simulink model "fblin_singletrack_schlacher"  (R2021a)
settings: Solver=ode45  StartTime=0.0  StopTime=20  RelTol=1e-3
PostLoadFcn:
  | clear all;
  | 
  | lf  = 0.1368;
  | lr  = 0.1232;
  | m  = 1.9;
  | mu = 0.385;
  | Cf = 50.13;
  | Cr = 122.05;
  | J = 0.029;
  | 
  | V0 = 1;
  | Vxp0 = 1;
  | Vxpf = 5;
  | Vyp0 = 0;
  | Vypf = 1;
settings Model: Creator=l_lan  LastModifiedBy=bascetta
settings SolverCC: MaxConsecutiveZCs=10000  MaxConsecutiveMinStep=1000
settings DataIOCC: SaveOutput=off  SignalLogging=off  DSMLogging=off  SaveTime=off  ReturnWorkspaceOutputs=off

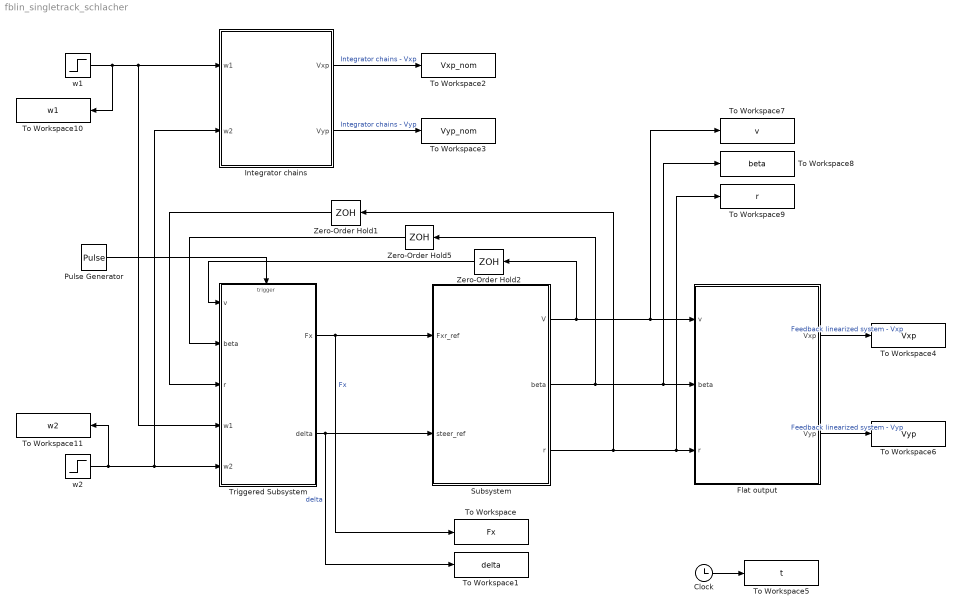
== system fblin_singletrack_schlacher ==
  Clock : Clock
  Flat output : Subsystem
  Integrator chains : Subsystem
  Pulse Generator : DiscretePulseGenerator  PulseType=Time based  Period=0.01  PulseWidth=50
  Subsystem : Subsystem
  To Workspace : ToWorkspace  VariableName=Fx  SampleTime=0.001
      settings: Save2DSignal=2-D array (concatenate along first dimension)
  To Workspace1 : ToWorkspace  VariableName=delta  SampleTime=0.001
      settings: Save2DSignal=2-D array (concatenate along first dimension)
  To Workspace10 : ToWorkspace  VariableName=w1  SampleTime=0.001
      settings: Save2DSignal=2-D array (concatenate along first dimension)
  To Workspace11 : ToWorkspace  VariableName=w2  SampleTime=0.001
      settings: Save2DSignal=2-D array (concatenate along first dimension)
  To Workspace2 : ToWorkspace  VariableName=Vxp_nom  SampleTime=0.001
      settings: Save2DSignal=2-D array (concatenate along first dimension)
  To Workspace3 : ToWorkspace  VariableName=Vyp_nom  SampleTime=0.001
      settings: Save2DSignal=2-D array (concatenate along first dimension)
  To Workspace4 : ToWorkspace  VariableName=Vxp  SampleTime=0.001
      settings: Save2DSignal=2-D array (concatenate along first dimension)
  To Workspace5 : ToWorkspace  VariableName=t  SampleTime=0.001
      settings: Save2DSignal=2-D array (concatenate along first dimension)
  To Workspace6 : ToWorkspace  VariableName=Vyp  SampleTime=0.001
      settings: Save2DSignal=2-D array (concatenate along first dimension)
  To Workspace7 : ToWorkspace  VariableName=v  SampleTime=0.001
      settings: Save2DSignal=2-D array (concatenate along first dimension)
  To Workspace8 : ToWorkspace  VariableName=beta  SampleTime=0.001
      settings: Save2DSignal=2-D array (concatenate along first dimension)
  To Workspace9 : ToWorkspace  VariableName=r  SampleTime=0.001
      settings: Save2DSignal=2-D array (concatenate along first dimension)
  Triggered Subsystem : Subsystem  TreatAsAtomicUnit=on
  Zero-Order Hold1 : ZeroOrderHold  SampleTime=0.01
  Zero-Order Hold2 : ZeroOrderHold  SampleTime=0.01
  Zero-Order Hold5 : ZeroOrderHold  SampleTime=0.01
  w1 : Step  Before=Vxp0  After=Vxpf  SampleTime=0
  w2 : Step  Time=5  Before=Vyp0  After=Vypf  SampleTime=0
  wires:
  Subsystem/3(r) -> Flat output/3(r), To Workspace9/1, Zero-Order Hold1/1
  Integrator chains/1(Vxp) -> To Workspace2/1  "Integrator chains - Vxp"
  w1/1 -> To Workspace10/1, Triggered Subsystem/4(w1), Integrator chains/1(w1)
  w2/1 -> To Workspace11/1, Integrator chains/2(w2), Triggered Subsystem/5(w2)
  Flat output/2(Vyp) -> To Workspace6/1  "Feedback linearized system - Vyp"
  Integrator chains/2(Vyp) -> To Workspace3/1  "Integrator chains - Vyp"
  Flat output/1(Vxp) -> To Workspace4/1  "Feedback linearized system - Vxp"
  Clock/1 -> To Workspace5/1
  Subsystem/2(beta) -> Zero-Order Hold5/1, Flat output/2(beta), To Workspace8/1
  Pulse Generator/1 -> Triggered Subsystem/Trigger
  Triggered Subsystem/1(Fx) -> Subsystem/1(Fxr_ref), To Workspace/1  "Fx"
  Triggered Subsystem/2(delta) -> Subsystem/2(steer_ref), To Workspace1/1  "delta"
  Zero-Order Hold1/1 -> Triggered Subsystem/3(r)
  Zero-Order Hold2/1 -> Triggered Subsystem/1(v)
  Zero-Order Hold5/1 -> Triggered Subsystem/2(beta)
  Subsystem/1(V) -> To Workspace7/1, Flat output/1(v), Zero-Order Hold2/1

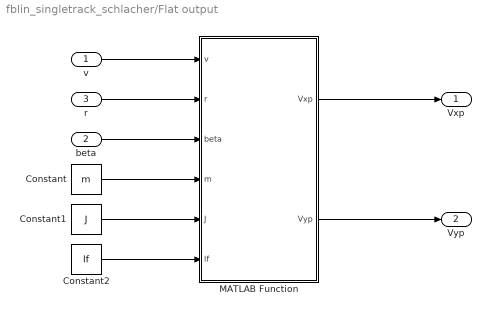
== system fblin_singletrack_schlacher/Flat output ==
  v : Inport
  beta : Inport  Port=2
  r : Inport  Port=3
  Constant : Constant  Value=m
  Constant1 : Constant  Value=J
  Constant2 : Constant  Value=lf
  MATLAB Function : MATLAB Function  TreatAsAtomicUnit=on
  Vxp : Outport
  Vyp : Outport  Port=2
  wires:
  beta/1 -> MATLAB Function/3(beta)
  r/1 -> MATLAB Function/2(r)
  v/1 -> MATLAB Function/1(v)
  Constant1/1 -> MATLAB Function/5(J)
  Constant/1 -> MATLAB Function/4(m)
  Constant2/1 -> MATLAB Function/6(lf)
  MATLAB Function/2(Vyp) -> Vyp/1
  MATLAB Function/1(Vxp) -> Vxp/1

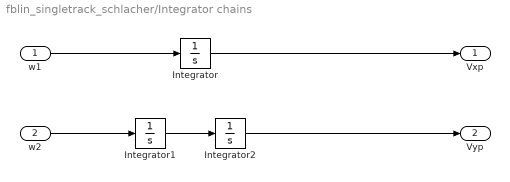
== system fblin_singletrack_schlacher/Integrator chains ==
  w1 : Inport
  w2 : Inport  Port=2
  Integrator : Integrator  InitialCondition=V0
  Integrator1 : Integrator
  Integrator2 : Integrator
  Vxp : Outport
  Vyp : Outport  Port=2
  wires:
  Integrator/1 -> Vxp/1
  Integrator1/1 -> Integrator2/1
  Integrator2/1 -> Vyp/1
  w2/1 -> Integrator1/1
  w1/1 -> Integrator/1

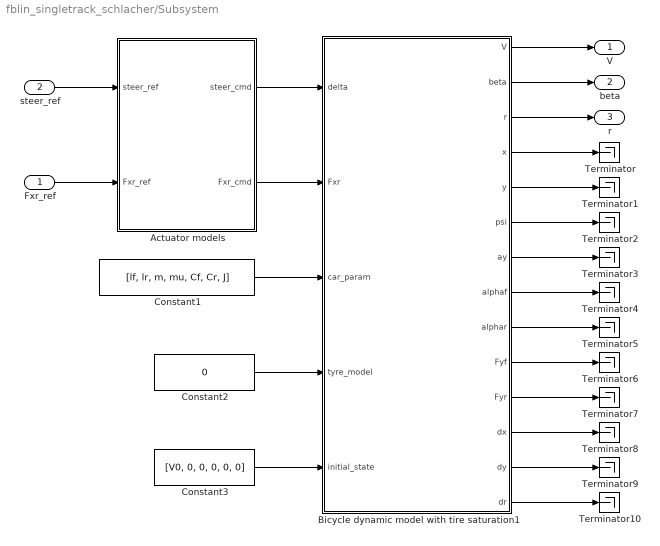
== system fblin_singletrack_schlacher/Subsystem ==
  Fxr_ref : Inport
  steer_ref : Inport  Port=2
  Actuator models : Subsystem  mask{mu_steer=1.0, wn_steer=87.62, csi_steer=0.75, tau_steer=0.055, steer_initial=0.0, mu_force=5.1282, wn_force=1000, csi_force=0.9, tau_force=0.0001, force_initial=0}
      mask prompts: mu_steer "Gain"; wn_steer "Natural frequency"; csi_steer "Damping"; tau_steer "Delay"; steer_initial "Initial value"; mu_force "Gain"; wn_force "Natural frequency"; csi_force "Damping"; tau_force "Delay"; force_initial "Initial value"
      mask DialogControl Container3 Prompt: Steer actuator parameters
      mask DialogControl Container4 Prompt: Speed actuator parameters
  Bicycle dynamic model with tire saturation1 : Subsystem
  Constant1 : Constant  Value=[lf, lr, m, mu, Cf, Cr, J]
  Constant2 : Constant  Value=0
  Constant3 : Constant  Value=[V0, 0, 0, 0, 0, 0]
  Terminator{,1..10} (11 alike) : Terminator
  V : Outport
  beta : Outport  Port=2
  r : Outport  Port=3
  wires:
  Constant2/1 -> Bicycle dynamic model with tire saturation1/4(tyre_model)
  Constant1/1 -> Bicycle dynamic model with tire saturation1/3(car_param)
  steer_ref/1 -> Actuator models/1(steer_ref)
  Actuator models/2(Fxr_cmd) -> Bicycle dynamic model with tire saturation1/2(Fxr)
  Fxr_ref/1 -> Actuator models/2(Fxr_ref)
  Actuator models/1(steer_cmd) -> Bicycle dynamic model with tire saturation1/1(delta)
  Constant3/1 -> Bicycle dynamic model with tire saturation1/5("initial_state ")
  Bicycle dynamic model with tire saturation1/3(r) -> r/1
  Bicycle dynamic model with tire saturation1/2(beta) -> beta/1
  Bicycle dynamic model with tire saturation1/1(V) -> V/1
  Bicycle dynamic model with tire saturation1/4(x) -> Terminator/1
  Bicycle dynamic model with tire saturation1/5(y) -> Terminator1/1
  Bicycle dynamic model with tire saturation1/6(psi) -> Terminator2/1
  Bicycle dynamic model with tire saturation1/7(ay) -> Terminator3/1
  Bicycle dynamic model with tire saturation1/8(alphaf) -> Terminator4/1
  Bicycle dynamic model with tire saturation1/9(alphar) -> Terminator5/1
  Bicycle dynamic model with tire saturation1/10(Fyf) -> Terminator6/1
  Bicycle dynamic model with tire saturation1/11(Fyr) -> Terminator7/1
  Bicycle dynamic model with tire saturation1/12(dx) -> Terminator8/1
  Bicycle dynamic model with tire saturation1/13(dy) -> Terminator9/1
  Bicycle dynamic model with tire saturation1/14(dr) -> Terminator10/1

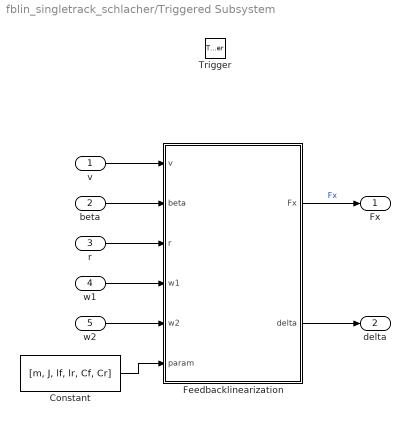
== system fblin_singletrack_schlacher/Triggered Subsystem ==
  v : Inport
  beta : Inport  Port=2
  r : Inport  Port=3
  w1 : Inport  Port=4
  w2 : Inport  Port=5
  Trigger : TriggerPort  VariantControl=(inherit)
  Constant : Constant  Value=[m, J, lf, lr, Cf, Cr]
  Feedbacklinearization : MATLAB Function  TreatAsAtomicUnit=on
  Fx : Outport
  delta : Outport  Port=2
  wires:
  Constant/1 -> Feedbacklinearization/6(param)
  v/1 -> Feedbacklinearization/1(v)
  beta/1 -> Feedbacklinearization/2(beta)
  r/1 -> Feedbacklinearization/3(r)
  w1/1 -> Feedbacklinearization/4(w1)
  w2/1 -> Feedbacklinearization/5(w2)
  Feedbacklinearization/2(delta) -> delta/1
  Feedbacklinearization/1(Fx) -> Fx/1  "Fx"

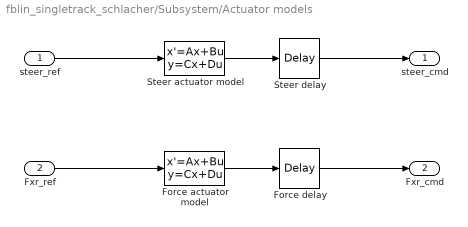
== system fblin_singletrack_schlacher/Subsystem/Actuator models ==
  steer_ref : Inport
  Fxr_ref : Inport  Port=2
  Force actuator model : StateSpace  A=[0, 1; -wn_force^2, -2*csi_force*wn_force]  B=[0; mu_force*wn_force^2]  C=[1, 0]  D=0  InitialCondition=[force_initial, 0]
  Force delay : TransportDelay  DelayTime=tau_force  InitialOutput=force_initial
  Steer actuator model : StateSpace  A=[0, 1; -wn_steer^2, -2*csi_steer*wn_steer]  B=[0; mu_steer*wn_steer^2]  C=[1, 0]  D=0  InitialCondition=[steer_initial, 0]
  Steer delay : TransportDelay  DelayTime=tau_steer  InitialOutput=steer_initial
  steer_cmd : Outport
  Fxr_cmd : Outport  Port=2
  wires:
  Fxr_ref/1 -> Force actuator model/1
  Steer actuator model/1 -> Steer delay/1
  Force actuator model/1 -> Force delay/1
  steer_ref/1 -> Steer actuator model/1
  Steer delay/1 -> steer_cmd/1
  Force delay/1 -> Fxr_cmd/1

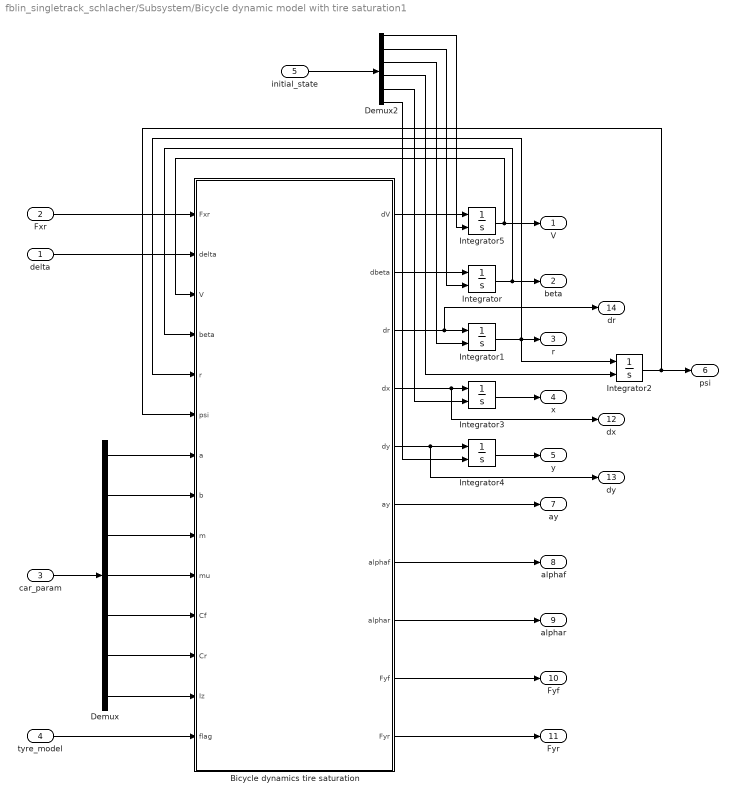
== system fblin_singletrack_schlacher/Subsystem/Bicycle dynamic model with tire saturation1 ==
  delta : Inport
  Fxr : Inport  Port=2
  car_param : Inport  Port=3
  tyre_model : Inport  Port=4
  "initial_state " : Inport  Port=5
  Bicycle dynamics tire saturation : MATLAB Function  TreatAsAtomicUnit=on
  Demux : Demux  Outputs=7
  Demux2 : Demux  Outputs=6
  Integrator{,1..5} (6 alike) : Integrator  InitialConditionSource=external
  V : Outport
  beta : Outport  Port=2
  r : Outport  Port=3
  x : Outport  Port=4
  y : Outport  Port=5
  psi : Outport  Port=6
  ay : Outport  Port=7
  alphaf : Outport  Port=8
  alphar : Outport  Port=9
  Fyf : Outport  Port=10
  Fyr : Outport  Port=11
  dx : Outport  Port=12
  dy : Outport  Port=13
  dr : Outport  Port=14
  wires:
  Fxr/1 -> Bicycle dynamics tire saturation/1(Fxr)
  delta/1 -> Bicycle dynamics tire saturation/2(delta)
  Bicycle dynamics tire saturation/2(dbeta) -> Integrator/1
  Bicycle dynamics tire saturation/3(dr) -> dr/1, Integrator1/1
  Integrator/1 -> beta/1, Bicycle dynamics tire saturation/4(beta)
  Integrator1/1 -> r/1, Integrator2/1, Bicycle dynamics tire saturation/5(r)
  Bicycle dynamics tire saturation/6(ay) -> ay/1
  Bicycle dynamics tire saturation/7(alphaf) -> alphaf/1
  Bicycle dynamics tire saturation/8(alphar) -> alphar/1
  Bicycle dynamics tire saturation/9(Fyf) -> Fyf/1
  Bicycle dynamics tire saturation/10(Fyr) -> Fyr/1
  car_param/1 -> Demux/1
  Demux/1 -> Bicycle dynamics tire saturation/7(a)
  Demux/2 -> Bicycle dynamics tire saturation/8(b)
  Demux/3 -> Bicycle dynamics tire saturation/9(m)
  Demux/4 -> Bicycle dynamics tire saturation/10(mu)
  "initial_state "/1 -> Demux2/1
  tyre_model/1 -> Bicycle dynamics tire saturation/14(flag)
  Demux/5 -> Bicycle dynamics tire saturation/11(Cf)
  Demux/6 -> Bicycle dynamics tire saturation/12(Cr)
  Demux/7 -> Bicycle dynamics tire saturation/13(Iz)
  Bicycle dynamics tire saturation/4(dx) -> Integrator3/1, dx/1
  Bicycle dynamics tire saturation/5(dy) -> Integrator4/1, dy/1
  Integrator3/1 -> x/1
  Integrator4/1 -> y/1
  Integrator2/1 -> Bicycle dynamics tire saturation/6(psi), psi/1
  Integrator5/1 -> V/1, Bicycle dynamics tire saturation/3(V)
  Demux2/1 -> Integrator5/2
  Bicycle dynamics tire saturation/1(dV) -> Integrator5/1
  Demux2/2 -> Integrator/2
  Demux2/3 -> Integrator1/2
  Demux2/4 -> Integrator2/2
  Demux2/5 -> Integrator3/2
  Demux2/6 -> Integrator4/2

== matlab function fblin_singletrack_schlacher/Subsystem/Bicycle dynamic model with tire saturation1/Bicycle dynamics tire saturation ==
  data: dV output; dbeta output; Fxr input; dr output; dx output; dy output; delta input; V input; beta input; r input; psi input; a input; b input; m input; mu input; Cf input; Cr input; Iz input; ay output; alphaf output; alphar output; Fyf output; Fyr output; flag input
function [dV,dbeta,dr,dx,dy,ay,alphaf,alphar,Fyf,Fyr]  = bicycle_dynamics(Fxr, delta, V, beta, r, psi, a, b, m, mu, Cf, Cr, Iz, flag)

Fzf = m*9.81*b/(a+b);
Fzr = m*9.81*a/(a+b);

if (abs(V*cos(beta))<=0.01)
    alphaf = 0;
    alphar = 0;
else
    alphaf = (V*sin(beta)+a*r)/(V*cos(beta))-delta;
    alphar = (V*sin(beta)-b*r)/(V*cos(beta));
end

zf = tan(alphaf);
zr = tan(alphar);

zf_sl = 3*mu*Fzf/Cf;
zr_sl = 3*mu*Fzr/Cr;

switch flag
    case 0 % Linear tyre model
        Fyf = -Cf*alphaf;
        Fyr = -Cr*alphar;
    case 1 % Fiala model with saturation
        if (abs(zf)<zf_sl)
            Fyf = Cf*zf*(-1+abs(zf)/zf_sl-zf^2/(3*zf_sl^2));
        else
            Fyf = -mu*Fzf*sign(alphaf);
        end
        if (abs(zr)<zr_sl)
            Fyr = Cr*zr*(-1+abs(zr)/zr_sl-zr^2/(3*zr_sl^2));
        else
            Fyr = -mu*Fzr*sign(alphar);
        end
    case 2 % Fiala model without saturation
        Fyf = Cf*zf*(-1+abs(zf)/zf_sl-zf^2/(3*zf_sl^2));
        Fyr = Cr*zr*(-1+abs(zr)/zr_sl-zr^2/(3*zr_sl^2));
    otherwise
        Fyf = 0;
        Fyr = 0;
end

dV    = (Fyf*(sin(beta)-cos(beta)*delta)+Fyr*sin(beta)+Fxr*cos(beta))/m;
dbeta = (Fyf*(cos(beta)+sin(beta)*delta)+Fyr*cos(beta)-Fxr*sin(beta))/(m*V)-r;
dr    = (a*Fyf-b*Fyr)/Iz;

ay    = (sin(beta)*dV+V*(cos(beta)^2-sin(beta)^2)/cos(beta)*dbeta)+r*V*cos(beta);

R_psi = [cos(psi), -sin(psi); sin(psi), cos(psi)];
dx  = R_psi(1,1:2)*[V*cos(beta); V*sin(beta)];
dy  = R_psi(2,1:2)*[V*cos(beta); V*sin(beta)];

== matlab function fblin_singletrack_schlacher/Triggered Subsystem/Feedbacklinearization ==
  data: v input; beta input; r input; w1 input; w2 input; Fx output; delta output; param input
function [Fx, delta] = fblin(v, beta, r, w1, w2, param)
m  = param(1);
J  = param(2);
lf = param(3);
lr = param(4);
Cf = param(5);
Cr = param(6);

l = (lf+lr)/(m*lf);
F = -(lf*v)/J*cos(beta)+(Cr*l)./(J*m*v*cos(beta))*(lf*lr*m-J);
R = (lr*v)/J*cos(beta)-(Cr*l)./(J*m*v*cos(beta))*(J+m*lr^2);
H = -r*w1+(Cr*l)./(v*cos(beta)).^2*(v*w1*sin(beta)-lr*r*w1-v^2*r*sin(beta)^2+r*v^2);
 
Fry   = Cr*(lr*r-v*sin(beta))./(v*cos(beta));        
delta = (w2-Fry*R-H)./(F*Cf)+(v*sin(beta)+lf*r)./(v*cos(beta));
Ffy   = Cf*(delta-(v*sin(beta)+lf*r)./(v*cos(beta)));     
Fx    = m*w1+Ffy*delta-v*r*m*sin(beta);

== matlab function fblin_singletrack_schlacher/Flat output/MATLAB Function ==
  data: v input; Vxp output; r input; beta input; m input; J input; lf input; Vyp output
function [Vxp,Vyp] = z_tranform(v,r,beta,m,J,lf)

Vxp = v*cos(beta);
Vyp = v*sin(beta)-J/(m*lf)*r;
